simulink model "zadatak1"  (R2018a)
settings: Solver=VariableStepAuto  StartTime=0.0  StopTime=1  RelTol=1e-3
undefined symbols (not defined in the file or in its folder): G, k, q, Rp, Rs
libraries: simulink x2
settings Model: Creator=User  LastModifiedBy=User

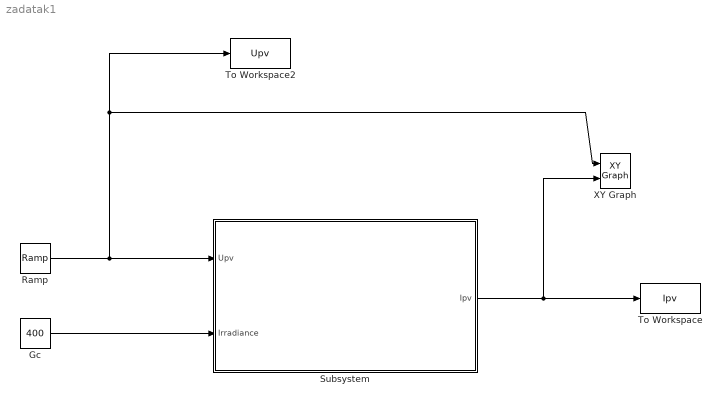
== system zadatak1 ==
  Gc : Constant  Value=400
  Ramp : simulink/Sources/Ramp  slope=0.7  start=0  InitialOutput=0
  Subsystem : Subsystem
  To Workspace : ToWorkspace  VariableName=Ipv  SampleTime=-1
  To Workspace2 : ToWorkspace  VariableName=Upv  SampleTime=-1
  XY Graph : simulink/Sinks/XY Graph  xmin=0  xmax=0.6  ymin=0  ymax=1.2  st=-1
  wires:
  Subsystem/1(Ipv) -> XY Graph/2, To Workspace/1
  Gc/1 -> Subsystem/2(Irradiance)
  Ramp/1 -> To Workspace2/1, XY Graph/1, Subsystem/1(Upv)

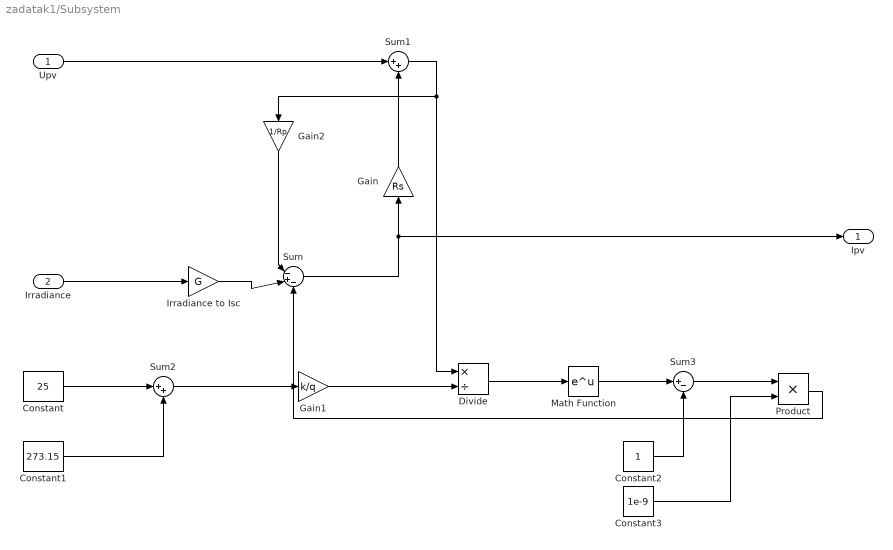
== system zadatak1/Subsystem ==
  Upv : Inport
  Irradiance : Inport  Port=2
  Constant : Constant  Value=25
  Constant1 : Constant  Value=273.15
  Constant2 : Constant
  Constant3 : Constant  Value=1e-9
  Divide : Product  Inputs=*/
  Gain : Gain  Gain=Rs
  Gain1 : Gain  Gain=k/q
  Gain2 : Gain  Gain=1/Rp
  "Irradiance to Isc " : Gain  Gain=G
  Math Function : Math  SaturateOnIntegerOverflow=on
  Product : Product
  Sum : Sum  Inputs=|-+-
  Sum1 : Sum  Inputs=|++
  Sum2 : Sum  Inputs=|++
  Sum3 : Sum  Inputs=|+-
  Ipv : Outport
  wires:
  Irradiance/1 -> "Irradiance to Isc "/1
  "Irradiance to Isc "/1 -> Sum/2
  Upv/1 -> Sum1/1
  Sum/1 -> Ipv/1, Gain/1
  Gain/1 -> Sum1/2
  Constant/1 -> Sum2/1
  Constant1/1 -> Sum2/2
  Sum2/1 -> Gain1/1
  Gain1/1 -> Divide/2
  Sum1/1 -> Gain2/1, Divide/1
  Gain2/1 -> Sum/1
  Divide/1 -> Math Function/1
  Math Function/1 -> Sum3/1
  Constant2/1 -> Sum3/2
  Sum3/1 -> Product/1
  Constant3/1 -> Product/2
  Product/1 -> Sum/3
